simulink model "pidcon1"  (R2020b)
settings: Solver=VariableStepAuto  StartTime=0.0  StopTime=10.0  RelTol=1e-3
settings Model: Creator=lalit  LastModifiedBy=lalit
settings DataIOCC: SaveOutput=off  SaveTime=off

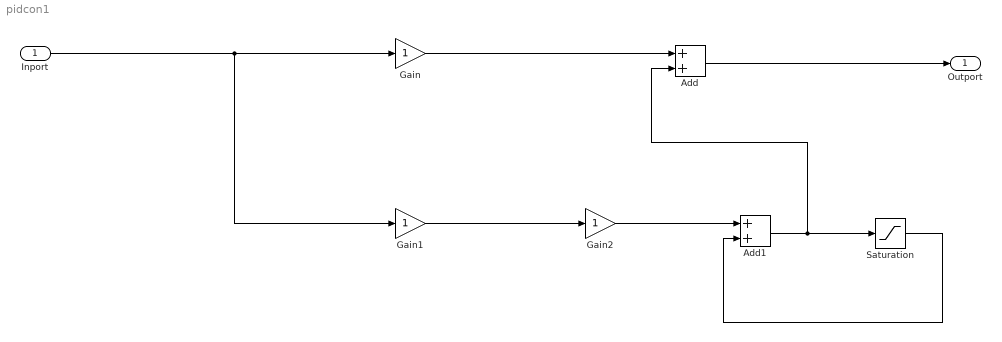
== system pidcon1 ==
  Inport : Inport  OutDataTypeStr=double  PortDimensions=1  SampleTime=0
  Add : Sum
  Add1 : Sum
  Gain : Gain
  Gain1 : Gain
  Gain2 : Gain
  Saturation : Saturate
  Outport : Outport  OutDataTypeStr=double  PortDimensions=1  SampleTime=0
  wires:
  Gain1/1 -> Gain2/1
  Saturation/1 -> Add1/2
  Gain/1 -> Add/1
  Add/1 -> Outport/1
  Add1/1 -> Saturation/1, Add/2
  Inport/1 -> Gain/1, Gain1/1
  Gain2/1 -> Add1/1
